simulink model "planta_1"  (Simulink 5.0)
settings: Solver=ode45  StartTime=0.0  StopTime=10.0  RelTol=1e-3
undefined symbols (not defined in the file): A0, g
settings Model: LastModifiedBy=pc1

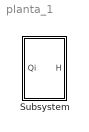
== system planta_1 ==
  Subsystem : Subsystem

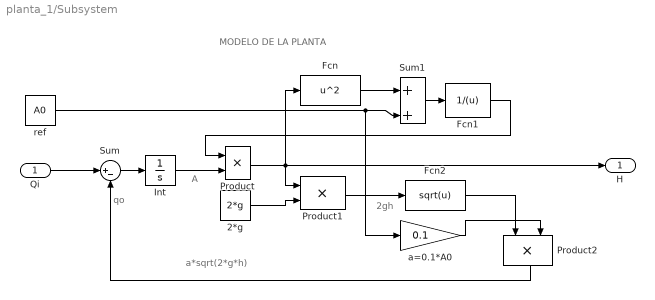
== system planta_1/Subsystem ==
  note: a*sqrt(2*g*h)
  note: A
  note: 2gh
  note: qo
  note: MODELO DE LA PLANTA
  Qi : Inport
  2*g : Constant  Value=2*g
  Fcn : Fcn  Expr=u^2
  Fcn1 : Fcn  Expr=1/(u)
  Fcn2 : Fcn  Expr=sqrt(u)
  Int : Integrator
  Product : Product  SaturateOnIntegerOverflow=on
  Product1 : Product  SaturateOnIntegerOverflow=on
  Product2 : Product  Orientation=down  SaturateOnIntegerOverflow=on
  Sum : Sum  Inputs=|+-  SaturateOnIntegerOverflow=on
  Sum1 : Sum  SaturateOnIntegerOverflow=on
  a=0.1*A0 : Gain  Gain=0.1  SaturateOnIntegerOverflow=on
  ref : Constant  Value=A0
  H : Outport
  wires:
  Int/1 -> Product/2
  Product/1 -> H/1, Fcn/1, Product1/1
  Qi/1 -> Sum/1
  Sum/1 -> Int/1
  Fcn/1 -> Sum1/1
  Sum1/1 -> Fcn1/1
  Fcn1/1 -> Product/1
  2*g/1 -> Product1/2
  Product1/1 -> Fcn2/1
  Fcn2/1 -> Product2/1
  a=0.1*A0/1 -> Product2/2
  ref/1 -> Sum1/2, a=0.1*A0/1
  Product2/1 -> Sum/2
